simulink model "pendulum_poleplace_sim"  (R2025b)
settings: Solver=VariableStepAuto  StartTime=0.0  StopTime=5  RelTol=1e-3
values from neighbouring files (symbols this model uses):
  A = [0 1 0 0 ... (first row only)    [correct.m]    (also in map.m; map12.m; map23.m; map32.m)
  B = [0 ... (first row only)    [correct.m]    (also in map.m = [0;1;0;4.9]; map12.m; map23.m; map32.m)
  K = place(A,B,p)    [map.m]    (also in map23.m)
  Nbar = -1/(Cr*(Acl\B))    [map.m]    (also in map23.m)
settings Model: Creator=fred  LastModifiedBy=fred

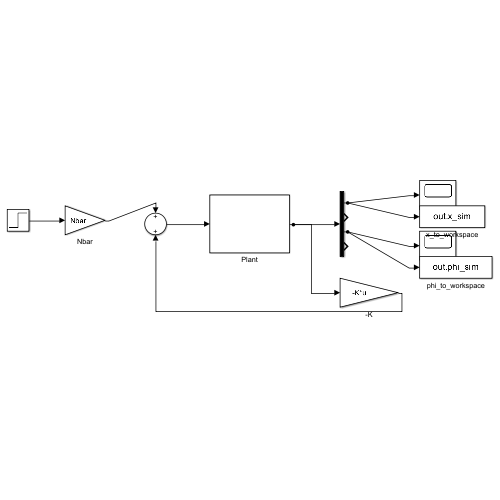
[thumbnail: Simulink's stored preview of the top-level diagram]
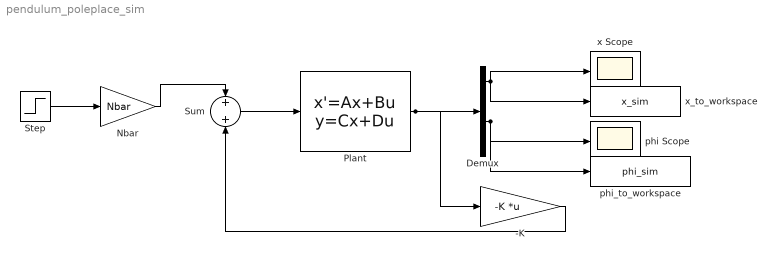
== system pendulum_poleplace_sim ==
  -K : Gain  Gain=-K  Multiplication=Matrix(K*u)
  Demux : Demux
  Nbar : Gain  Gain=Nbar
  Plant : StateSpace  A=A  B=B  C=eye(4)  D=zeros(4,1)  InitialCondition=0
  Step : Step  Time=0  After=0.1  SampleTime=0
  Sum : Sum
  phi Scope : Scope
  phi_to_workspace : ToWorkspace  VariableName=phi_sim  SaveFormat=Structure With Time  SampleTime=-1
  x Scope : Scope
  x_to_workspace : ToWorkspace  VariableName=x_sim  SaveFormat=Structure With Time  SampleTime=-1
  wires:
  Step/1 -> Nbar/1
  Nbar/1 -> Sum/1
  Sum/1 -> Plant/1
  Plant/1 -> Demux/1, -K/1
  -K/1 -> Sum/2
  Demux/1 -> x Scope/1, x_to_workspace/1
  Demux/3 -> phi Scope/1, phi_to_workspace/1
